simulink model "UnTanque"  (Simulink 5.0)
settings: Solver=ode5  StartTime=0.0  StopTime=Inf  FixedStep=0.125  MinStep=0.01  RelTol=1e-3
libraries: simulink x2
settings Model: LastModifiedBy=L10  RTWOptions="-aEnforceIntegerDowncast=1 -aExtMode=0 -aExtModeTesting=0 -aFoldNonRolledExpr=1 -aForceParamTrailComments=0 -aGenerateComments=1 -aGenerateReport=0 -aIgnoreCustomStorageClasses=1 -aIncDataTypeInIds=0 -aIncHierarchyInIds=0 -aInlineInvariantSignals=0 -aInlinedPrmAccess=\"Literals\" -aLocalBlockOutputs=1 -aLogVarNameModifier=\"rt_\" -aMaxRTWIdLen=31 -aPrefixModelToSubsysFcnNames=1 -aRTWVerbose=1 -aRollThreshold=5 -aShowEliminatedStatements=0"

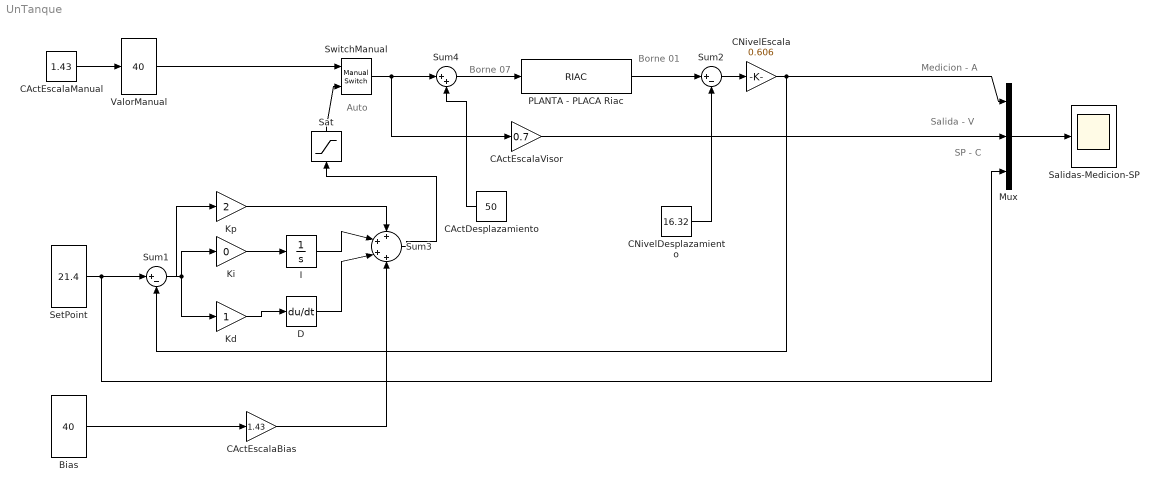
== system UnTanque ==
  note: Auto
  note: Medicion - A
  note: Salida - V
  note: SP - C
  note: Borne 07
  note: Borne 01
  Bias : Constant  Value=40  VectorParams1D=off
  CActDesplazamiento : Constant  Orientation=left  Value=50  VectorParams1D=off
  CActEscalaBias : Gain  Gain=1.43  SaturateOnIntegerOverflow=on
  CActEscalaManual : Constant  Value=1.43  VectorParams1D=off
  CActEscalaVisor : Gain  Gain=0.7  SaturateOnIntegerOverflow=on
  CNivelDesplazamiento : Constant  Value=16.32  VectorParams1D=off
  CNivelEscala : Gain  Gain=0.606  SaturateOnIntegerOverflow=on
  D : Derivative
  I : Integrator  LimitOutput=on  UpperSaturationLimit=180  LowerSaturationLimit=-180
  Kd : Gain  SaturateOnIntegerOverflow=on
  Ki : Gain  Gain=0  SaturateOnIntegerOverflow=on
  Kp : Gain  Gain=2  SaturateOnIntegerOverflow=on
  Mux : Mux  Inputs=3
  PLANTA - PLACA Riac : S-Function  FunctionName=RIAC
  Salidas-Medicion-SP : Scope
      settings: TimeRange=300  YMin=0  YMax=100
  Sat : Saturate  Orientation=up  UpperLimit=180  LowerLimit=0
  SetPoint : Constant  Value=21.4  VectorParams1D=off
  Sum1 : Sum  Inputs=|+-  SaturateOnIntegerOverflow=on
  Sum2 : Sum  Inputs=|+-  SaturateOnIntegerOverflow=on
  Sum3 : Sum  Inputs=++++  SaturateOnIntegerOverflow=on
  Sum4 : Sum  Inputs=|++  SaturateOnIntegerOverflow=on
  SwitchManual : simulink/Signal Routing/Manual Switch  sw=0  action=0
  ValorManual : simulink/Math Operations/Slider Gain  low=0  gain=40  high=100
  wires:
  Mux/1 -> Salidas-Medicion-SP/1
  ValorManual/1 -> SwitchManual/1
  SetPoint/1 -> Sum1/1, Mux/3
  Bias/1 -> CActEscalaBias/1
  Sat/1 -> SwitchManual/2
  PLANTA - PLACA Riac/1 -> Sum2/1
  Sum2/1 -> CNivelEscala/1
  CNivelEscala/1 -> Mux/1, Sum1/2
  CNivelDesplazamiento/1 -> Sum2/2
  SwitchManual/1 -> Sum4/1, CActEscalaVisor/1
  CActDesplazamiento/1 -> Sum4/2
  Sum4/1 -> PLANTA - PLACA Riac/1
  CActEscalaVisor/1 -> Mux/2
  CActEscalaManual/1 -> ValorManual/1
  Sum1/1 -> Kp/1, Ki/1, Kd/1
  Sum3/1 -> Sat/1
  CActEscalaBias/1 -> Sum3/4
  Ki/1 -> I/1
  I/1 -> Sum3/2
  Kp/1 -> Sum3/1
  Kd/1 -> D/1
  D/1 -> Sum3/3
